simulink library "Radiation_Divison"  (Simulink 8.2)
settings: Solver=ode45  StartTime=0.0  StopTime=10.0  RelTol=1e-3
settings Model: Creator=drhf  LastModifiedBy=drhf

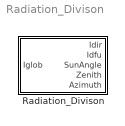
== system Radiation_Divison ==
  Radiation_Divison : Subsystem  mask(Radiation Division){latitude=51, longitude=-7, longitude0=-30}
      mask prompts: latitude "Latitude [-90;90], north positive"; longitude "Longitude  [-180;180], west positive"; longitude0 "reference longitude (timezone)"
      mask help:
      | Calculates the direct and diffusive radiation on the horizontal surface as parts of the global radiation.
      |
      | INPUT VECTOR:
      |   time      : real time or simulation time  [s]
      |   Iglob     : global radiation on horizontal surface (W/m²)
      |
      | OUTPUT VECTORS:
      |   Idir           : direct radiation (W/m²)
      |   Idfu          : diffusive radiation (W/m²)
      |   SunAngle
      |   Zenith
      |   Azimuth
      mask Help: web(fullfile(path_carnot('help'),'Radiation_Divison.html'),'-helpbrowser')

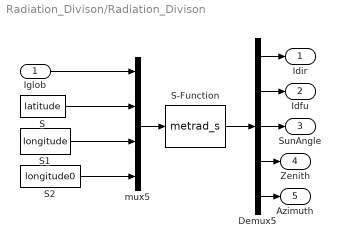
== system Radiation_Divison/Radiation_Divison ==
  Iglob : Inport
  Demux5 : Demux  Outputs=5
  S : Constant  Value=latitude
  S-Function : S-Function  FunctionName=metrad_s  EnableBusSupport=off
  S1 : Constant  Value=longitude
  S2 : Constant  Value=longitude0
  mux5 : Mux
  Idir : Outport
  Idfu : Outport  Port=2
  SunAngle : Outport  Port=3
  Zenith : Outport  Port=4
  Azimuth : Outport  Port=5
  wires:
  S2/1 -> mux5/4
  S1/1 -> mux5/3
  S/1 -> mux5/2
  Iglob/1 -> mux5/1
  mux5/1 -> S-Function/1
  S-Function/1 -> Demux5/1
  Demux5/1 -> Idir/1
  Demux5/2 -> Idfu/1
  Demux5/3 -> SunAngle/1
  Demux5/4 -> Zenith/1
  Demux5/5 -> Azimuth/1
